simulink model "Assignment1"  (R2020b)
settings: Solver=VariableStepAuto  StartTime=0.0  StopTime=10.0  RelTol=1e-3
values from neighbouring files (symbols this model uses):
  T = 1/((20*wc)/(2*pi))    (= 0.0010471975512)    [Assignment1.m]    (also in Assignment3.m = [1/(2.5*bw) 1/(10*bw) 1/(25*bw)]; Lecture15_DigitalLSF.m = 1 / ((25 * bandwidth(tf([10], [2 2 1])))); Lecture4_DiscretePID.m = 0.1)
settings Model: Creator=sebastian  LastModifiedBy=sebastian

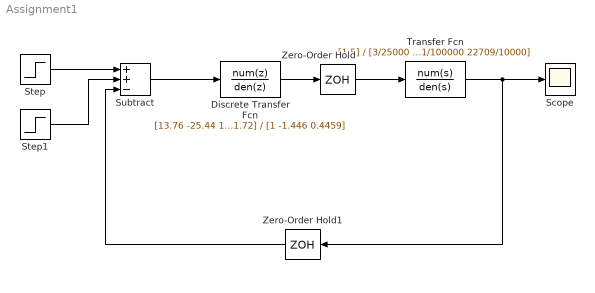
== system Assignment1 ==
  Discrete Transfer Fcn : DiscreteTransferFcn  Numerator=[13.76 -25.44 11.72]  Denominator=[1 -1.446 0.4459]
  Scope : Scope
  Step : Step  SampleTime=0
  Step1 : Step  Time=2  After=-1  SampleTime=0
  Subtract : Sum  Inputs=++-
  Transfer Fcn : TransferFcn  Numerator=[1.5]  Denominator=[3/25000 2291/100000 22709/10000]
  Zero-Order Hold : ZeroOrderHold  SampleTime=T
  Zero-Order Hold1 : ZeroOrderHold  SampleTime=T
  wires:
  Step/1 -> Subtract/1
  Subtract/1 -> Discrete Transfer Fcn/1
  Discrete Transfer Fcn/1 -> Zero-Order Hold/1
  Zero-Order Hold/1 -> Transfer Fcn/1
  Transfer Fcn/1 -> Zero-Order Hold1/1, Scope/1
  Zero-Order Hold1/1 -> Subtract/3
  Step1/1 -> Subtract/2
